simulink model "pid_1dof_linear_speed"  (R2017a)
settings: Solver=ode45  StartTime=0.0  StopTime=10  RelTol=1e-3
undefined symbols (not defined in the file): A, B, GoalPos, k_p, x0
libraries: simulink x1
settings Model: Creator=sansh  LastModifiedBy=rj2318

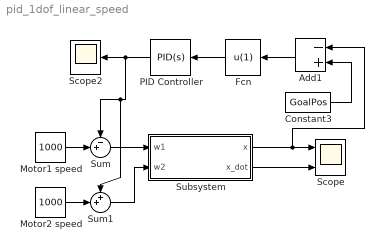
== system pid_1dof_linear_speed ==
  Add1 : Sum  Inputs=-+
  Constant3 : Constant  Value=GoalPos
  Fcn : Fcn  Expr=u(1)
  Motor1 speed : Constant  Value=1000
  Motor2 speed : Constant  Value=1000
  PID Controller : simulink/Continuous/PID Controller  Controller=PID  TimeDomain=Continuous-time  SampleTime=-1  IntegratorMethod=Forward Euler  FilterMethod=Forward Euler  Form=Parallel  UseFilter=on  ControllerParametersSource=internal  P=10  I=0.1  D=10  N=10  InitialConditionSource=internal  InitialConditionForIntegrator=0  InitialConditionForFilter=0  ExternalReset=none  LimitOutput=off  UpperSaturationLimit=inf  LowerSaturationLimit=-inf  LinearizeAsGain=on  AntiWindupMode=none  Kb=1  TrackingMode=off  Kt=1  PParamMin=[]  PParamMax=[]  IParamMin=[]  IParamMax=[]  DParamMin=[]  DParamMax=[]  NParamMin=[]  NParamMax=[]  KbParamMin=[]  KbParamMax=[]  KtParamMin=[]  KtParamMax=[]  POutMin=[]  POutMax=[]  IOutMin=[]  IOutMax=[]  DOutMin=[]  DOutMax=[]  NOutMin=[]  NOutMax=[]  KbOutMin=[]  KbOutMax=[]  KtOutMin=[]  KtOutMax=[]  IntegratorOutMin=[]  IntegratorOutMax=[]  FilterOutMin=[]  FilterOutMax=[]  SumOutMin=[]  SumOutMax=[]  SumI1OutMin=[]  SumI1OutMax=[]  SumI2OutMin=[]  SumI2OutMax=[]  SumI3OutMin=[]  SumI3OutMax=[]  SumDOutMin=[]  SumDOutMax=[]  SaturationOutMin=[]  SaturationOutMax=[]  IntegratorContinuousStateAttributes=''  IntegratorStateMustResolveToSignalObject=off  IntegratorRTWStateStorageClass=Auto  FilterContinuousStateAttributes=''  FilterStateMustResolveToSignalObject=off  FilterRTWStateStorageClass=Auto  DifferentiatorICPrevScaledInput=0  DifferentiatorOutMin=[]  DifferentiatorOutMax=[]
  Scope : Scope  NumInputPorts=2
  Scope2 : Scope
  Subsystem : Subsystem
  Sum : Sum  Inputs=-+|
  Sum1 : Sum  Inputs=++|
  wires:
  Constant3/1 -> Add1/2
  Subsystem/2(x_dot) -> Scope/2
  Subsystem/1(x) -> Add1/1, Scope/1
  Add1/1 -> Fcn/1
  Fcn/1 -> PID Controller/1
  Sum/1 -> Subsystem/1(w1)
  Motor2 speed/1 -> Sum1/2
  PID Controller/1 -> Sum/1, Sum1/1, Scope2/1
  Motor1 speed/1 -> Sum/2
  Sum1/1 -> Subsystem/2(w2)

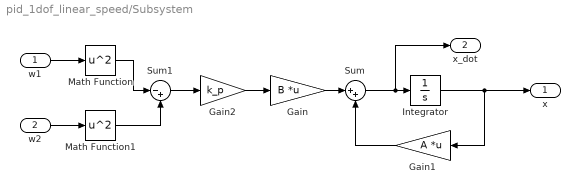
== system pid_1dof_linear_speed/Subsystem ==
  w1 : Inport
  w2 : Inport  Port=2
  Gain : Gain  Gain=B  Multiplication=Matrix(K*u)
  Gain1 : Gain  Gain=A  Multiplication=Matrix(K*u)
  Gain2 : Gain  Gain=k_p
  Integrator : Integrator  InitialCondition=x0
  Math Function : Math  Operator=square  SaturateOnIntegerOverflow=on
  Math Function1 : Math  Operator=square  SaturateOnIntegerOverflow=on
  Sum : Sum  Inputs=|++
  Sum1 : Sum  Inputs=|-+
  x : Outport
  x_dot : Outport  Port=2
  wires:
  Gain1/1 -> Sum/2
  Integrator/1 -> Gain1/1, x/1
  Sum/1 -> x_dot/1, Integrator/1
  Gain/1 -> Sum/1
  w2/1 -> Math Function1/1
  Gain2/1 -> Gain/1
  Sum1/1 -> Gain2/1
  Math Function/1 -> Sum1/1
  Math Function1/1 -> Sum1/2
  w1/1 -> Math Function/1
